simulink model "perfil_obstaculos"  (R2023b)
settings: Solver=VariableStepAuto  StartTime=0.0  StopTime=10.0  RelTol=1e-3
settings Model: Creator=Ferran  LastModifiedBy=Ferran

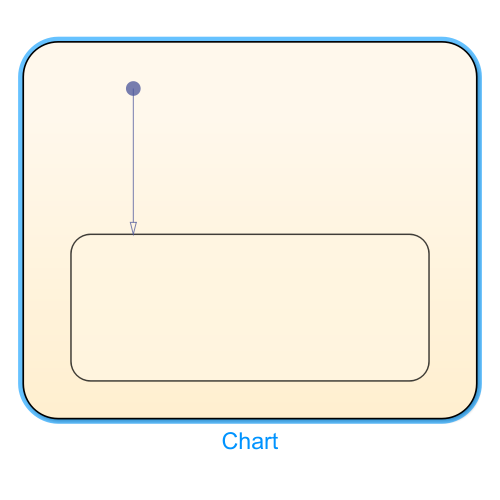
[thumbnail: Simulink's stored preview of the top-level diagram]
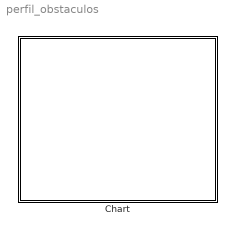
== system perfil_obstaculos ==
  Chart : Stateflow chart  TreatAsAtomicUnit=on

== stateflow chart perfil_obstaculos/Chart ==
  state ?
  (default) -> ?
